simulink model "DiodeRectifier_NPCInverter"  (R2020a)
settings: Solver=ode23t  StartTime=0.0  StopTime=0.25  MaxStep=10e-6  RelTol=1e-3
libraries: powerlib x51, simulink x6
settings Model: Creator=Matthew  LastModifiedBy=Matthew

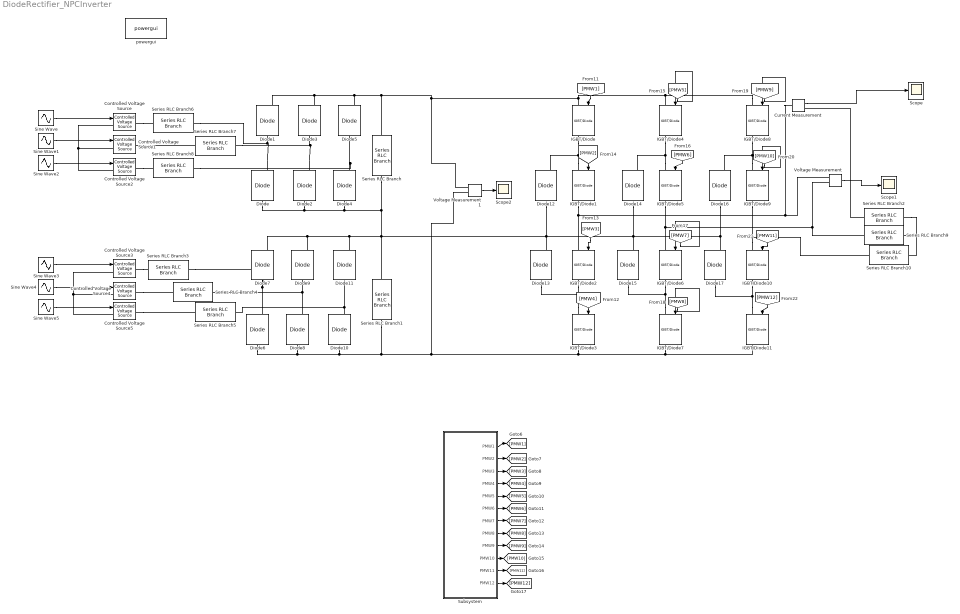
== system DiodeRectifier_NPCInverter ==
  Controlled Voltage Source{,1..5} (6 alike) : powerlib/Electrical Sources/Controlled Voltage Source  Initialize=on  Source_Type=AC  Amplitude=1900  Phase=0  Frequency=50  Measurements=None
  Current Measurement : powerlib/Measurements/Current Measurement  PhasorSimulation=off  OutputType=Complex  PSBequivalent=0
  Diode{,1..17} (18 alike) : powerlib/Power Electronics/Diode  Ron=0.001  Lon=0  Vf=0.8  IC=0  UseSnubber=0  Rs=500  Cs=250e-9  Measurements=on
  IGBT/Diode{,1..11} (12 alike) : powerlib/Power Electronics/IGBT//Diode  Ron=1e-3  Rs=1e5  Cs=inf  Measurements=on
  Scope : Scope
  Scope1 : Scope
  Scope2 : Scope
  Series RLC Branch : powerlib/Elements/Series RLC Branch  LConnTagsString=__new0  RConnTagsString=__new0  BranchType=C  Resistance=1e-3  Inductance=5600e-6  SetiL0=off  InitialCurrent=0  Capacitance=1000e-6  Setx0=off  InitialVoltage=0  Measurements=None
  Series RLC Branch1 : powerlib/Elements/Series RLC Branch  LConnTagsString=__new0  RConnTagsString=__new0  BranchType=C  Resistance=1e-3  Inductance=5600e-6  SetiL0=off  InitialCurrent=0  Capacitance=1000e-6  Setx0=off  InitialVoltage=0  Measurements=None
  Series RLC Branch10 : powerlib/Elements/Series RLC Branch  LConnTagsString=__new0  RConnTagsString=__new0  BranchType=RL  Resistance=100  Inductance=10e-3  SetiL0=off  InitialCurrent=0  Capacitance=1000e-6  Setx0=off  InitialVoltage=0  Measurements=None
  Series RLC Branch2 : powerlib/Elements/Series RLC Branch  LConnTagsString=__new0  RConnTagsString=__new0  BranchType=RL  Resistance=100  Inductance=10e-3  SetiL0=off  InitialCurrent=0  Capacitance=1000e-6  Setx0=off  InitialVoltage=0  Measurements=None
  Series RLC Branch{3..8} (6 alike) : powerlib/Elements/Series RLC Branch  LConnTagsString=__new0  RConnTagsString=__new0  BranchType=L  Resistance=1e-3  Inductance=3e-3  SetiL0=off  InitialCurrent=0  Capacitance=1000e-6  Setx0=off  InitialVoltage=0  Measurements=None
  Series RLC Branch9 : powerlib/Elements/Series RLC Branch  LConnTagsString=__new0  RConnTagsString=__new0  BranchType=RL  Resistance=100  Inductance=10e-3  SetiL0=off  InitialCurrent=0  Capacitance=1000e-6  Setx0=off  InitialVoltage=0  Measurements=None
  Sine Wave : Sin  Amplitude=1900*1.414  Frequency=2*pi*60  SampleTime=0
  Sine Wave1 : Sin  Amplitude=1900*1.414  Frequency=2*pi*60  Phase=-2*pi/3  SampleTime=0
  Sine Wave2 : Sin  Amplitude=1900*1.414  Frequency=2*pi*60  Phase=2*pi/3  SampleTime=0
  Sine Wave3 : Sin  Amplitude=1900*1.414  Frequency=2*pi*60  Phase=30/360*pi  SampleTime=0
  Sine Wave4 : Sin  Amplitude=1900*1.414  Frequency=2*pi*60  Phase=-2*pi/3+30/360*pi  SampleTime=0
  Sine Wave5 : Sin  Amplitude=1900*1.414  Frequency=2*pi*60  Phase=2*pi/3+30/360*pi  SampleTime=0
  Subsystem : Subsystem
  Voltage Measurement : powerlib/Measurements/Voltage Measurement  PhasorSimulation=off  OutputType=Complex  PSBequivalent=0
  Voltage Measurement1 : powerlib/Measurements/Voltage Measurement  PhasorSimulation=off  OutputType=Complex  PSBequivalent=0
  powergui : powerlib/powergui  Priority=1  SimulationMode=Discrete  SampleTime=10e-6  frequency=60  Iterations=50  frequencyindice=0  Pbase=100e6  ErrMax=1e-4  UnitsV=kV  UnitsW=MW  buscounter=0  FunctionMessages=off  echomessages=off  EnableUseOfTLC=off  CurrentSourceSwitches=off  DisableSnubberDevices=off  DisableRonSwitches=off  DisableVfSwitches=off  DisplayEquations=off  AutomaticDiscreteSolvers=off  SolverType=Tustin/Backward Euler (TBE)  Interpol=off  ExternalGateDelay=off  methode=off  Ts=100  x0status=blocks  SPID=on  SwTol=0  HookPort=off  NonlinearTolerance=1e-4  nMaxIteration=100  ContinueOnMaxIteration=off  RestoreLinks=warning  ResistiveCurrentMeasurement=off  Frange=[0:2:500]  Ylog=off  Xlog=on  ShowGrid=off  save=off  variable=ZData  structure=0  ZoomFFT=off  StartTime=0.0  cycles=1  DisplayStyle=1  fundamental=60  FreqAxis=off  MaxFrequency=1000  frequencyindicesteady=1  RmsSteady=1  display=off
  wires:
  Sine Wave/1 -> Controlled Voltage Source/1
  Sine Wave1/1 -> Controlled Voltage Source1/1
  Sine Wave2/1 -> Controlled Voltage Source2/1
  Sine Wave5/1 -> Controlled Voltage Source5/1
  Sine Wave4/1 -> Controlled Voltage Source4/1
  Sine Wave3/1 -> Controlled Voltage Source3/1
  Voltage Measurement1/1 -> Scope2/1
  Subsystem/8(PMW8) -> [PMW8]
  [PMW1] -> IGBT/Diode/1
  [PMW8] -> IGBT/Diode7/1
  Subsystem/11(PMW11) -> [PMW11]
  Subsystem/7(PMW7) -> [PMW7]
  Subsystem/12(PMW12) -> [PMW12]
  Subsystem/10(PMW10) -> [PMW10]
  Subsystem/6(PMW6) -> [PMW6]
  [PMW2] -> IGBT/Diode1/1
  [PMW6] -> IGBT/Diode5/1
  Subsystem/2(PMW2) -> [PMW2]
  [PMW4] -> IGBT/Diode3/1
  Subsystem/4(PMW4) -> [PMW4]
  [PMW3] -> IGBT/Diode2/1
  Subsystem/9(PMW9) -> [PMW9]
  Subsystem/5(PMW5) -> [PMW5]
  [PMW5] -> IGBT/Diode4/1
  Voltage Measurement/1 -> Scope1/1
  Current Measurement/1 -> Scope/1
  [PMW11] -> IGBT/Diode10/1
  [PMW9] -> IGBT/Diode8/1
  [PMW7] -> IGBT/Diode6/1
  [PMW12] -> IGBT/Diode11/1
  Subsystem/1(PMW1) -> [PMW1]
  Subsystem/3(PMW3) -> [PMW3]
  [PMW10] -> IGBT/Diode9/1
  connections:
  Controlled Voltage Source/RConn1 -- Series RLC Branch6/RConn1
  Controlled Voltage Source1/RConn1 -- Series RLC Branch7/RConn1
  Controlled Voltage Source2/RConn1 -- Series RLC Branch8/RConn1
  IGBT/Diode8/LConn1 -- IGBT/Diode/LConn1 -- Diode1/RConn1 -- Diode3/RConn1 -- Diode5/RConn1 -- Series RLC Branch/LConn1 -- Voltage Measurement1/LConn1 -- IGBT/Diode4/LConn1
  IGBT/Diode11/RConn1 -- IGBT/Diode7/RConn1 -- Diode6/LConn1 -- Diode8/LConn1 -- Diode10/LConn1 -- Series RLC Branch1/RConn1 -- Voltage Measurement1/LConn2 -- IGBT/Diode3/RConn1
  Diode6/RConn1 -- Series RLC Branch3/LConn1 -- Diode7/LConn1
  Controlled Voltage Source5/RConn1 -- Series RLC Branch5/RConn1
  Diode8/RConn1 -- Series RLC Branch4/LConn1 -- Diode9/LConn1
  Diode16/LConn1 -- Diode17/RConn1 -- Diode14/LConn1 -- Diode15/RConn1 -- Diode/LConn1 -- Diode2/LConn1 -- Diode4/LConn1 -- Series RLC Branch/RConn1 -- Series RLC Branch1/LConn1 -- Diode11/RConn1 -- Diode9/RConn1 -- Diode7/RConn1 -- Diode12/LConn1 -- Diode13/RConn1
  Controlled Voltage Source2/LConn1 -- Controlled Voltage Source1/LConn1 -- Controlled Voltage Source/LConn1
  Controlled Voltage Source5/LConn1 -- Controlled Voltage Source3/LConn1 -- Controlled Voltage Source4/LConn1
  Controlled Voltage Source3/RConn1 -- Series RLC Branch3/RConn1
  Controlled Voltage Source4/RConn1 -- Series RLC Branch4/RConn1
  Series RLC Branch5/LConn1 -- Diode11/LConn1 -- Diode10/RConn1
  Series RLC Branch6/LConn1 -- Diode/RConn1 -- Diode1/LConn1
  Series RLC Branch7/LConn1 -- Diode2/RConn1 -- Diode3/LConn1
  Series RLC Branch8/LConn1 -- Diode5/LConn1 -- Diode4/RConn1
  Series RLC Branch2/RConn1 -- Current Measurement/RConn1
  IGBT/Diode10/LConn1 -- IGBT/Diode9/RConn1 -- Series RLC Branch10/RConn1
  IGBT/Diode5/LConn1 -- IGBT/Diode4/RConn1 -- Diode14/RConn1
  IGBT/Diode7/LConn1 -- IGBT/Diode6/RConn1 -- Diode15/LConn1
  IGBT/Diode3/LConn1 -- IGBT/Diode2/RConn1 -- Diode13/LConn1
  IGBT/Diode1/LConn1 -- IGBT/Diode/RConn1 -- Diode12/RConn1
  Voltage Measurement/LConn2 -- IGBT/Diode5/RConn1 -- IGBT/Diode6/LConn1 -- Series RLC Branch9/RConn1
  IGBT/Diode11/LConn1 -- IGBT/Diode10/RConn1 -- Diode17/LConn1
  IGBT/Diode9/LConn1 -- IGBT/Diode8/RConn1 -- Diode16/RConn1
  Series RLC Branch9/LConn1 -- Series RLC Branch2/LConn1 -- Series RLC Branch10/LConn1
  Current Measurement/LConn1 -- Voltage Measurement/LConn1 -- IGBT/Diode1/RConn1 -- IGBT/Diode2/LConn1

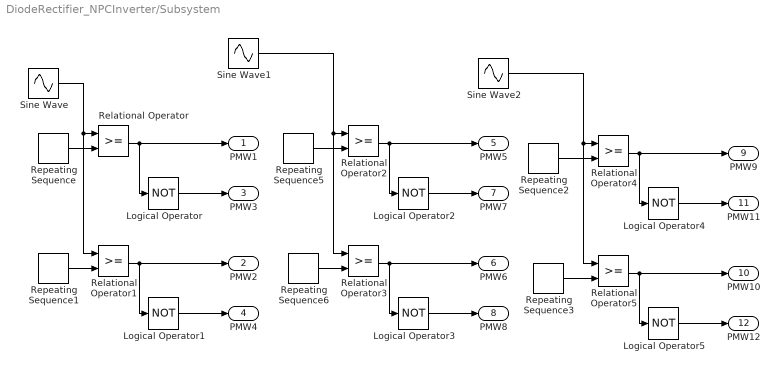
== system DiodeRectifier_NPCInverter/Subsystem ==
  Logical Operator{,1..5} (6 alike) : Logic  Operator=NOT  AllPortsSameDT=off  OutDataTypeStr=boolean
  Relational Operator{,1..5} (6 alike) : RelationalOperator  OutDataTypeStr=boolean  RndMeth=Simplest
  Repeating Sequence : simulink/Sources/Repeating Sequence  rep_seq_t=[0 1 2]*1/(20e3)  rep_seq_y=[0 1 0]
  Repeating Sequence1 : simulink/Sources/Repeating Sequence  rep_seq_t=[0 1 2]*1/(20e3)  rep_seq_y=[-1 0 -1]
  Repeating Sequence2 : simulink/Sources/Repeating Sequence  rep_seq_t=[0 1 2]*1/(20e3)  rep_seq_y=[0 1 0]
  Repeating Sequence3 : simulink/Sources/Repeating Sequence  rep_seq_t=[0 1 2]*1/(20e3)  rep_seq_y=[-1 0 -1]
  Repeating Sequence5 : simulink/Sources/Repeating Sequence  rep_seq_t=[0 1 2]*1/(20e3)  rep_seq_y=[0 1 0]
  Repeating Sequence6 : simulink/Sources/Repeating Sequence  rep_seq_t=[0 1 2]*1/(20e3)  rep_seq_y=[-1 0 -1]
  Sine Wave : Sin  Frequency=2*pi*60  SampleTime=0
  Sine Wave1 : Sin  Frequency=2*pi*60  Phase=-2*pi/3  SampleTime=0
  Sine Wave2 : Sin  Frequency=2*pi*60  Phase=2*pi/3  SampleTime=0
  PMW1 : Outport
  PMW2 : Outport  Port=2
  PMW3 : Outport  Port=3
  PMW4 : Outport  Port=4
  PMW5 : Outport  Port=5
  PMW6 : Outport  Port=6
  PMW7 : Outport  Port=7
  PMW8 : Outport  Port=8
  PMW9 : Outport  Port=9
  PMW10 : Outport  Port=10
  PMW11 : Outport  Port=11
  PMW12 : Outport  Port=12
  wires:
  Relational Operator2/1 -> PMW5/1, Logical Operator2/1
  Logical Operator2/1 -> PMW7/1
  Relational Operator4/1 -> PMW9/1, Logical Operator4/1
  Relational Operator3/1 -> PMW6/1, Logical Operator3/1
  Logical Operator4/1 -> PMW11/1
  Relational Operator1/1 -> PMW2/1, Logical Operator1/1
  Logical Operator3/1 -> PMW8/1
  Relational Operator/1 -> PMW1/1, Logical Operator/1
  Repeating Sequence/1 -> Relational Operator/2
  Repeating Sequence2/1 -> Relational Operator4/2
  Relational Operator5/1 -> PMW10/1, Logical Operator5/1
  Sine Wave2/1 -> Relational Operator5/1, Relational Operator4/1
  Logical Operator5/1 -> PMW12/1
  Sine Wave/1 -> Relational Operator/1, Relational Operator1/1
  Sine Wave1/1 -> Relational Operator2/1, Relational Operator3/1
  Repeating Sequence3/1 -> Relational Operator5/2
  Repeating Sequence1/1 -> Relational Operator1/2
  Repeating Sequence5/1 -> Relational Operator2/2
  Logical Operator1/1 -> PMW4/1
  Logical Operator/1 -> PMW3/1
  Repeating Sequence6/1 -> Relational Operator3/2
